simulink model "bsp_nxt_ultrasonic"  (R2019a)
settings: Solver=FixedStepAuto  StartTime=0.0  StopTime=inf  FixedStep=Ts  RelTol=1e-3  EnableMultiTasking=on
libraries: BrickPiSimSubLib_initreset x2, BrickPiSimSubLib_getsensor x1
settings Model: SimulationMode=external  Creator=uk008555  LastModifiedBy=uk008555
settings SolverCC: PositivePriorityOrder=on
settings OptimizationCC: EnhancedBackFolding=on  PassReuseOutputArgsAs=Individual arguments  MaxStackSize=64  OptimizeBlockOrder=speed  DifferentSizesBufferReuse=on  OptimizationCustomize=off
settings DebuggingCC: ParameterTunabilityLossMsg=error
settings HardwareCC: ProdBitPerPointer=32  ProdBitPerSizeT=32  ProdBitPerPtrDiffT=32  ProdLargestAtomicInteger=Long  ProdLargestAtomicFloat=Double  ProdWordSize=32  ProdLongLongMode=on  ProdHWDeviceType=ARM Compatible->ARM Cortex
settings SFSimCC: MATLABDynamicMemAlloc=off
settings RTWCC: SystemTargetFile=ert.tlc  HardwareBoard=Raspberry Pi  TLCOptions="-aInlineSetEventsForThisBaseRateFcn=TLC_FALSE -aSuppressMultiTaskScheduler=TLC_FALSE  -aRateBasedStepFcn=0"  TemplateMakefile=ert_default_tmf  GenerateReport=on  Toolchain=GNU GCC Raspberry Pi  BuildConfiguration=Faster Runs  IncludeHyperlinkInReport=on  LaunchReport=on  GenerateTraceInfo=on  GenerateTraceReport=on  GenerateTraceReportSl=on  GenerateTraceReportSf=on  GenerateTraceReportEml=on
settings CodeAppCC: ForceParamTrailComments=on  IgnoreCustomStorageClasses=off  OperatorAnnotations=on  SimulinkDataObjDesc=on  SFDataObjDesc=on  InsertBlockDesc=on
settings ERTTargetCC: SupportVariableSizeSignals=on

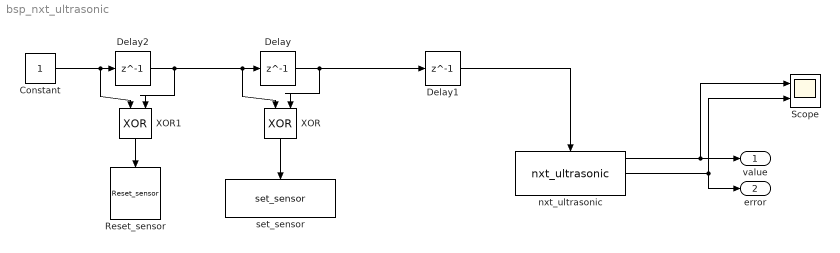
== system bsp_nxt_ultrasonic ==
  Constant : Constant
  Delay : Delay  DelayLength=1
  Delay1 : Delay  DelayLength=1
  Delay2 : Delay  DelayLength=1
  Reset_sensor : BrickPiSimSubLib_initreset/Reset_sensor  Port1_Val=off  Port2_Val=off  Port3_Val=off  Port4_Val=on
      settings: SourceProductName=Simulink Support Package for BrickPi
  Scope : Scope  NumInputPorts=2
  XOR : Logic  Operator=XOR  IconShape=distinctive  AllPortsSameDT=off  OutDataTypeStr=boolean
  XOR1 : Logic  Operator=XOR  IconShape=distinctive  AllPortsSameDT=off  OutDataTypeStr=boolean
  nxt_ultrasonic : BrickPiSimSubLib_getsensor/nxt_ultrasonic  Port_Val=4
      settings: SourceProductName=Simulink Support Package for BrickPi
  set_sensor : BrickPiSimSubLib_initreset/set_sensor  Type_Val=NXT Ultrasonic  Port_Val=4
      settings: SourceProductName=Simulink Support Package for BrickPi
  value : Outport
  error : Outport  Port=2
  wires:
  nxt_ultrasonic/1 -> Scope/1, value/1
  nxt_ultrasonic/2 -> error/1, Scope/2
  Delay/1 -> XOR/2, Delay1/1
  Delay1/1 -> nxt_ultrasonic/Enable
  XOR/1 -> set_sensor/Enable
  Constant/1 -> XOR1/1, Delay2/1
  Delay2/1 -> XOR1/2, XOR/1, Delay/1
  XOR1/1 -> Reset_sensor/Enable
